simulink model "glideslope_and_flare"  (R2017a)
settings: Solver=VariableStepAuto  StartTime=0.0  StopTime=140  RelTol=1e-3
values from neighbouring files (symbols this model uses):
  A = A_longitude_lo([1,2,3,4,5],[1,2,3,4,5])    [glideslope_and_flare_control.m]
  alpha_trim = trim_state_lin(8)*180/pi    [glideslope_and_flare_control.m]
  B = A_longitude_lo([1,2,3,4,5],[6,7])    [glideslope_and_flare_control.m]
  C = C_longitude_lo([1,2,3,4,5],[1,2,3,4,5])    [glideslope_and_flare_control.m]
  D = C_longitude_lo([1,2,3,4,5],[6,7])    [glideslope_and_flare_control.m]
  glide_slope_ref = 3    [glideslope_and_flare_control.m]
  hf = x2*tan(glide_slope_ref*pi/180)+10    [glideslope_and_flare_control.m]
  ht_trim = trim_state_lin(3)    [glideslope_and_flare_control.m]
  runway_altitude = 3000    [glideslope_and_flare_control.m]
  tau = x1/(flaretouchdowntime*velocity_trim-velocity_trim*cos(glide_slope_ref*pi/180))    [glideslope_and_flare_control.m]
  theta_trim = trim_state_lin(5)*180/pi    [glideslope_and_flare_control.m]
  time_interception = 10    [glideslope_and_flare_control.m]
  trim_control_lin = trim_control_lo    [FindF16Dynamics.m]
  trim_thrust_lin = trim_thrust_lo    [FindF16Dynamics.m]
  velocity_trim = trim_state_lin(7)    [glideslope_and_flare_control.m]
undefined symbols (not defined in the file or in its folder): magnitude
libraries: simulink x8
settings Model: Creator=chatto  LastModifiedBy=chatto

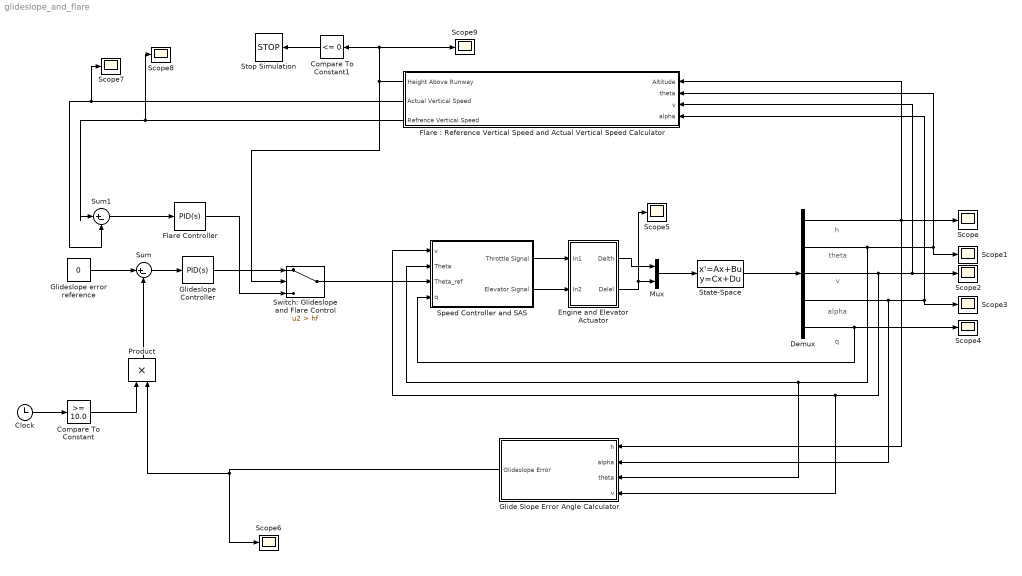
== system glideslope_and_flare ==
  note: alpha
  note: v
  note: theta
  note: h
  note: q
  Clock : Clock
  Compare To Constant : simulink/Logic and Bit Operations/Compare To Constant  relop=>=  const=10.0  OutDataTypeStr=boolean
  Compare To Constant1 : simulink/Logic and Bit Operations/Compare To Constant  relop=<=  const=0  OutDataTypeStr=boolean
  Demux : Demux  Outputs=5
  Engine and Elevator Actuator : Subsystem
  "Flare : Reference Vertical Speed and Actual Vertical Speed Calculator" : Subsystem
  Flare Controller : simulink/Continuous/PID Controller  Controller=PID  TimeDomain=Continuous-time  SampleTime=-1  IntegratorMethod=Forward Euler  FilterMethod=Forward Euler  Form=Parallel  UseFilter=on  ControllerParametersSource=internal  P=0.33  I=0  D=0.33  N=100  InitialConditionSource=internal  InitialConditionForIntegrator=0  InitialConditionForFilter=0  ExternalReset=none  LimitOutput=off  UpperSaturationLimit=inf  LowerSaturationLimit=-inf  LinearizeAsGain=on  AntiWindupMode=none  Kb=1  TrackingMode=off  Kt=1  PParamMin=[]  PParamMax=[]  IParamMin=[]  IParamMax=[]  DParamMin=[]  DParamMax=[]  NParamMin=[]  NParamMax=[]  KbParamMin=[]  KbParamMax=[]  KtParamMin=[]  KtParamMax=[]  POutMin=[]  POutMax=[]  IOutMin=[]  IOutMax=[]  DOutMin=[]  DOutMax=[]  NOutMin=[]  NOutMax=[]  KbOutMin=[]  KbOutMax=[]  KtOutMin=[]  KtOutMax=[]  IntegratorOutMin=[]  IntegratorOutMax=[]  FilterOutMin=[]  FilterOutMax=[]  SumOutMin=[]  SumOutMax=[]  SumI1OutMin=[]  SumI1OutMax=[]  SumI2OutMin=[]  SumI2OutMax=[]  SumI3OutMin=[]  SumI3OutMax=[]  SumDOutMin=[]  SumDOutMax=[]  SaturationOutMin=[]  SaturationOutMax=[]  IntegratorContinuousStateAttributes=''  IntegratorStateMustResolveToSignalObject=off  IntegratorRTWStateStorageClass=Auto  FilterContinuousStateAttributes=''  FilterStateMustResolveToSignalObject=off  FilterRTWStateStorageClass=Auto  DifferentiatorICPrevScaledInput=0  DifferentiatorOutMin=[]  DifferentiatorOutMax=[]  InitialConditionSetting=State (most efficient)
  Glide Slope Error Angle Calculator : Subsystem
  Glideslope Controller : simulink/Continuous/PID Controller  Controller=PID  TimeDomain=Continuous-time  SampleTime=-1  IntegratorMethod=Forward Euler  FilterMethod=Forward Euler  Form=Parallel  UseFilter=on  ControllerParametersSource=internal  P=80  I=8  D=100  N=100  InitialConditionSource=internal  InitialConditionForIntegrator=0  InitialConditionForFilter=0  ExternalReset=none  LimitOutput=off  UpperSaturationLimit=inf  LowerSaturationLimit=-inf  LinearizeAsGain=on  AntiWindupMode=none  Kb=1  TrackingMode=off  Kt=1  PParamMin=[]  PParamMax=[]  IParamMin=[]  IParamMax=[]  DParamMin=[]  DParamMax=[]  NParamMin=[]  NParamMax=[]  KbParamMin=[]  KbParamMax=[]  KtParamMin=[]  KtParamMax=[]  POutMin=[]  POutMax=[]  IOutMin=[]  IOutMax=[]  DOutMin=[]  DOutMax=[]  NOutMin=[]  NOutMax=[]  KbOutMin=[]  KbOutMax=[]  KtOutMin=[]  KtOutMax=[]  IntegratorOutMin=[]  IntegratorOutMax=[]  FilterOutMin=[]  FilterOutMax=[]  SumOutMin=[]  SumOutMax=[]  SumI1OutMin=[]  SumI1OutMax=[]  SumI2OutMin=[]  SumI2OutMax=[]  SumI3OutMin=[]  SumI3OutMax=[]  SumDOutMin=[]  SumDOutMax=[]  SaturationOutMin=[]  SaturationOutMax=[]  IntegratorContinuousStateAttributes=''  IntegratorStateMustResolveToSignalObject=off  IntegratorRTWStateStorageClass=Auto  FilterContinuousStateAttributes=''  FilterStateMustResolveToSignalObject=off  FilterRTWStateStorageClass=Auto  DifferentiatorICPrevScaledInput=0  DifferentiatorOutMin=[]  DifferentiatorOutMax=[]  InitialConditionSetting=State (most efficient)
  Glideslope error reference : Constant  Value=0
  Mux : Mux  Inputs=2
  Product : Product
  Scope{,1..9} (10 alike) : Scope
  Speed Controller and SAS : Subsystem
  State-Space : StateSpace  A=A  B=B  C=C  D=D  X0=0
  Stop Simulation : Stop
  Sum : Sum  Inputs=|+-
  Sum1 : Sum  Inputs=|+-
  Switch: Glideslope and Flare Control : Switch  Criteria=u2 > Threshold  Threshold=hf
  wires:
  Mux/1 -> State-Space/1
  State-Space/1 -> Demux/1
  Engine and Elevator Actuator/1(Delth) -> Mux/1
  Engine and Elevator Actuator/2(Delel) -> Scope5/1, Mux/2
  Sum/1 -> Glideslope Controller/1
  Speed Controller and SAS/1(Throttle Signal) -> Engine and Elevator Actuator/1(In1)
  Speed Controller and SAS/2(Elevator Signal) -> Engine and Elevator Actuator/2(In2)
  Demux/5 -> Speed Controller and SAS/4(q), Scope4/1
  Glideslope error reference/1 -> Sum/1
  Glideslope Controller/1 -> Switch: Glideslope and Flare Control/1
  Clock/1 -> Compare To Constant/1
  Compare To Constant/1 -> Product/1
  Product/1 -> Sum/2
  Glide Slope Error Angle Calculator/1(Glideslope Error) -> Scope6/1, Product/2
  Demux/1 -> Glide Slope Error Angle Calculator/1(h), Scope/1, "Flare : Reference Vertical Speed and Actual Vertical Speed Calculator"/1(Altitude)
  Demux/3 -> "Flare : Reference Vertical Speed and Actual Vertical Speed Calculator"/3(v), Scope2/1, Glide Slope Error Angle Calculator/4(v), Speed Controller and SAS/1(v)
  Demux/2 -> "Flare : Reference Vertical Speed and Actual Vertical Speed Calculator"/2(theta), Scope1/1, Glide Slope Error Angle Calculator/3(theta), Speed Controller and SAS/2(Theta)
  Demux/4 -> Glide Slope Error Angle Calculator/2(alpha), "Flare : Reference Vertical Speed and Actual Vertical Speed Calculator"/4(alpha), Scope3/1
  "Flare : Reference Vertical Speed and Actual Vertical Speed Calculator"/3(Refrence Vertical Speed) -> Scope8/1, Sum1/1
  "Flare : Reference Vertical Speed and Actual Vertical Speed Calculator"/2(Actual Vertical Speed) -> Scope7/1, Sum1/2
  Compare To Constant1/1 -> Stop Simulation/1
  Sum1/1 -> Flare Controller/1
  Switch: Glideslope and Flare Control/1 -> Speed Controller and SAS/3(Theta_ref)
  Flare Controller/1 -> Switch: Glideslope and Flare Control/3
  "Flare : Reference Vertical Speed and Actual Vertical Speed Calculator"/1(Height Above Runway) -> Scope9/1, Compare To Constant1/1, Switch: Glideslope and Flare Control/2

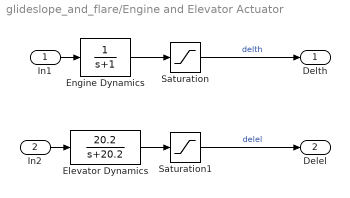
== system glideslope_and_flare/Engine and Elevator Actuator ==
  In1 : Inport
  In2 : Inport  Port=2
  Elevator Dynamics : TransferFcn  Numerator=[20.2]  Denominator=[1 20.2]
  Engine Dynamics : TransferFcn  Denominator=[1 1]
  Saturation : Saturate  UpperLimit=19000-trim_thrust_lin  LowerLimit=1000-trim_thrust_lin
  Saturation1 : Saturate  UpperLimit=25-trim_control_lin(1)  LowerLimit=-25-trim_control_lin(1)
  Delth : Outport
  Delel : Outport  Port=2
  wires:
  Saturation1/1 -> Delel/1  "delel"
  In1/1 -> Engine Dynamics/1
  In2/1 -> Elevator Dynamics/1
  Elevator Dynamics/1 -> Saturation1/1
  Engine Dynamics/1 -> Saturation/1
  Saturation/1 -> Delth/1  "delth"

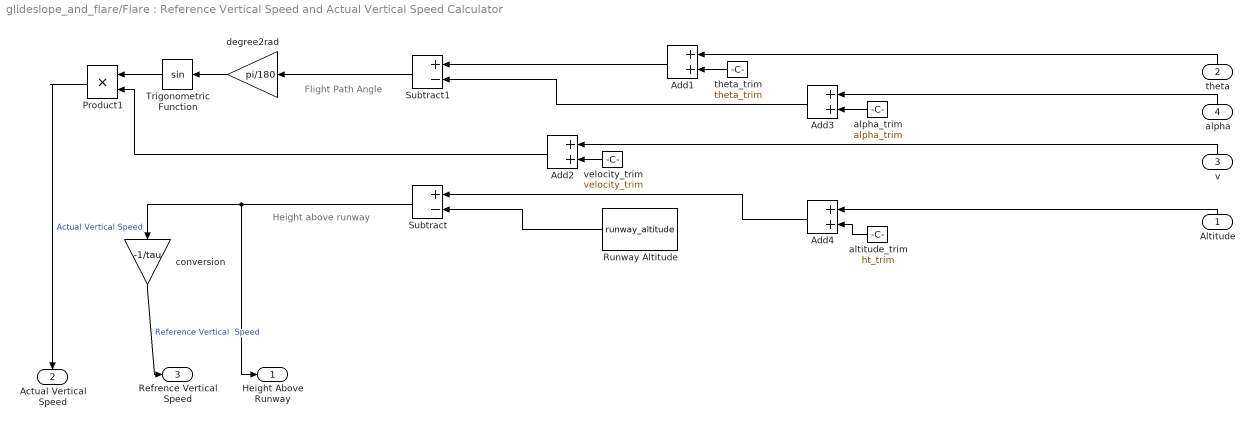
== system glideslope_and_flare/Flare : Reference Vertical Speed and Actual Vertical Speed Calculator ==
  note: Flight Path Angle
  note: Height above runway
  Altitude : Inport
  theta : Inport  Port=2
  v : Inport  Port=3
  alpha : Inport  Port=4
  Add{1..4} (4 alike) : Sum
  Product1 : Product
  Runway Altitude : Constant  Value=runway_altitude
  Subtract : Sum  Inputs=+-
  Subtract1 : Sum  Inputs=+-
  Trigonometric Function : Trigonometry
  alpha_trim : Constant  Value=alpha_trim
  altitude_trim : Constant  Value=ht_trim
  conversion : Gain  Gain=-1/tau
  degree2rad : Gain  Gain=pi/180
  theta_trim : Constant  Value=theta_trim
  velocity_trim : Constant  Value=velocity_trim
  Height Above Runway : Outport
  Actual Vertical Speed : Outport  Port=2
  Refrence Vertical Speed : Outport  Port=3
  wires:
  alpha_trim/1 -> Add3/2
  Runway Altitude/1 -> Subtract/2
  Trigonometric Function/1 -> Product1/1
  Altitude/1 -> Add4/1
  Add4/1 -> Subtract/1
  Add3/1 -> Subtract1/2
  alpha/1 -> Add3/1
  theta/1 -> Add1/1
  Product1/1 -> Actual Vertical Speed/1  "Actual Vertical Speed"
  theta_trim/1 -> Add1/2
  degree2rad/1 -> Trigonometric Function/1
  Add2/1 -> Product1/2
  v/1 -> Add2/1
  Add1/1 -> Subtract1/1
  altitude_trim/1 -> Add4/2
  conversion/1 -> Refrence Vertical Speed/1  "Reference Vertical  Speed"
  Subtract1/1 -> degree2rad/1
  velocity_trim/1 -> Add2/2
  Subtract/1 -> Height Above Runway/1, conversion/1

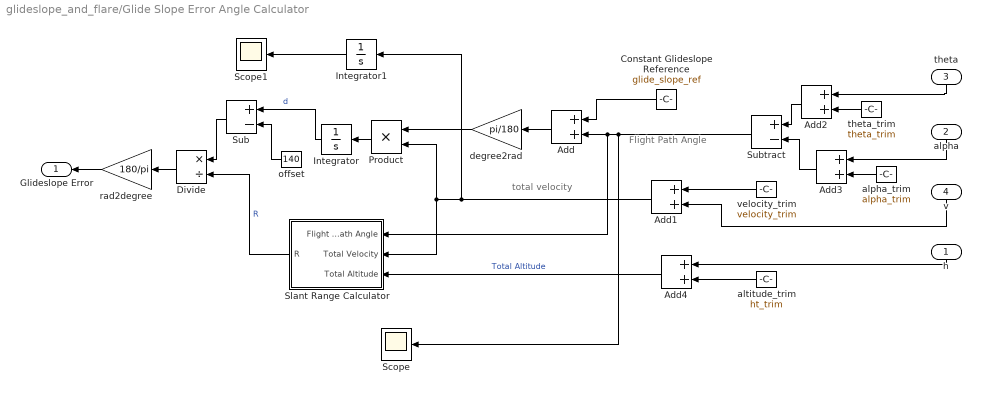
== system glideslope_and_flare/Glide Slope Error Angle Calculator ==
  note: total velocity
  note: Flight Path Angle
  h : Inport
  alpha : Inport  Port=2
  theta : Inport  Port=3
  v : Inport  Port=4
  Add{,1..4} (5 alike) : Sum
  Constant Glideslope Reference : Constant  Value=glide_slope_ref
  Divide : Product  Inputs=*/
  Integrator : Integrator
  Integrator1 : Integrator
  Product : Product
  Scope : Scope
  Scope1 : Scope
  Slant Range Calculator : Subsystem
  Sub : Sum  Inputs=+-
  Subtract : Sum  Inputs=+-
  alpha_trim : Constant  Value=alpha_trim
  altitude_trim : Constant  Value=ht_trim
  degree2rad : Gain  Gain=pi/180
  offset : Constant  Value=140
  rad2degree : Gain  Gain=180/pi
  theta_trim : Constant  Value=theta_trim
  velocity_trim : Constant  Value=velocity_trim
  Glideslope Error : Outport
  wires:
  altitude_trim/1 -> Add4/2
  Divide/1 -> rad2degree/1
  velocity_trim/1 -> Add1/1
  v/1 -> Add1/2
  alpha_trim/1 -> Add3/2
  Add2/1 -> Subtract/1
  theta_trim/1 -> Add2/2
  Add4/1 -> Slant Range Calculator/3(Total Altitude)  "Total Altitude"
  Constant Glideslope Reference/1 -> Add/1
  alpha/1 -> Add3/1
  h/1 -> Add4/1
  theta/1 -> Add2/1
  Add/1 -> degree2rad/1
  Add3/1 -> Subtract/2
  Integrator/1 -> Sub/1  "d"
  degree2rad/1 -> Product/1
  Product/1 -> Integrator/1
  Slant Range Calculator/1(R) -> Divide/2  "R"
  rad2degree/1 -> Glideslope Error/1
  Add1/1 -> Integrator1/1, Product/2, Slant Range Calculator/2(Total Velocity)
  Subtract/1 -> Slant Range Calculator/1(Flight Path Angle), Add/2, Scope/1
  offset/1 -> Sub/2
  Sub/1 -> Divide/1
  Integrator1/1 -> Scope1/1

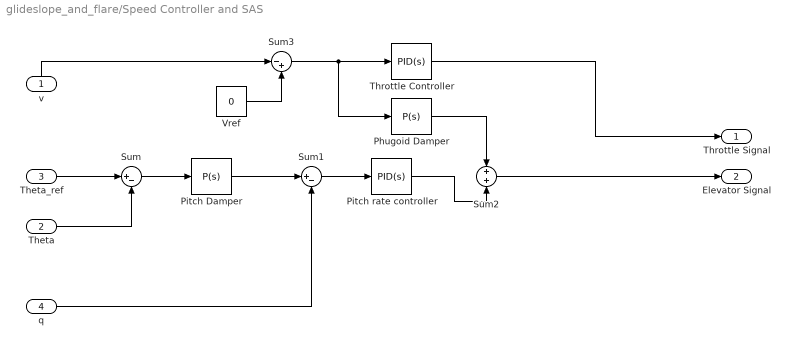
== system glideslope_and_flare/Speed Controller and SAS ==
  v : Inport
  Theta : Inport  Port=2
  Theta_ref : Inport  Port=3
  q : Inport  Port=4
  Phugoid Damper : simulink/Continuous/PID Controller  Controller=P  TimeDomain=Continuous-time  SampleTime=-1  IntegratorMethod=Forward Euler  FilterMethod=Forward Euler  Form=Parallel  UseFilter=on  ControllerParametersSource=internal  P=0.05  I=0.001  D=0.5  N=100  InitialConditionSource=internal  InitialConditionForIntegrator=0  InitialConditionForFilter=0  ExternalReset=none  LimitOutput=off  UpperSaturationLimit=inf  LowerSaturationLimit=-inf  LinearizeAsGain=on  AntiWindupMode=none  Kb=1  TrackingMode=off  Kt=1  PParamMin=[]  PParamMax=[]  IParamMin=[]  IParamMax=[]  DParamMin=[]  DParamMax=[]  NParamMin=[]  NParamMax=[]  KbParamMin=[]  KbParamMax=[]  KtParamMin=[]  KtParamMax=[]  POutMin=[]  POutMax=[]  IOutMin=[]  IOutMax=[]  DOutMin=[]  DOutMax=[]  NOutMin=[]  NOutMax=[]  KbOutMin=[]  KbOutMax=[]  KtOutMin=[]  KtOutMax=[]  IntegratorOutMin=[]  IntegratorOutMax=[]  FilterOutMin=[]  FilterOutMax=[]  SumOutMin=[]  SumOutMax=[]  SumI1OutMin=[]  SumI1OutMax=[]  SumI2OutMin=[]  SumI2OutMax=[]  SumI3OutMin=[]  SumI3OutMax=[]  SumDOutMin=[]  SumDOutMax=[]  SaturationOutMin=[]  SaturationOutMax=[]  IntegratorContinuousStateAttributes=''  IntegratorStateMustResolveToSignalObject=off  IntegratorRTWStateStorageClass=Auto  FilterContinuousStateAttributes=''  FilterStateMustResolveToSignalObject=off  FilterRTWStateStorageClass=Auto  DifferentiatorICPrevScaledInput=0  DifferentiatorOutMin=[]  DifferentiatorOutMax=[]  InitialConditionSetting=State (most efficient)
  Pitch Damper : simulink/Continuous/PID Controller  Controller=P  TimeDomain=Continuous-time  SampleTime=-1  IntegratorMethod=Forward Euler  FilterMethod=Forward Euler  Form=Parallel  UseFilter=on  ControllerParametersSource=internal  P=0.5  I=0  D=0  N=100  InitialConditionSource=internal  InitialConditionForIntegrator=0  InitialConditionForFilter=0  ExternalReset=none  LimitOutput=off  UpperSaturationLimit=inf  LowerSaturationLimit=-inf  LinearizeAsGain=on  AntiWindupMode=none  Kb=1  TrackingMode=off  Kt=1  PParamMin=[]  PParamMax=[]  IParamMin=[]  IParamMax=[]  DParamMin=[]  DParamMax=[]  NParamMin=[]  NParamMax=[]  KbParamMin=[]  KbParamMax=[]  KtParamMin=[]  KtParamMax=[]  POutMin=[]  POutMax=[]  IOutMin=[]  IOutMax=[]  DOutMin=[]  DOutMax=[]  NOutMin=[]  NOutMax=[]  KbOutMin=[]  KbOutMax=[]  KtOutMin=[]  KtOutMax=[]  IntegratorOutMin=[]  IntegratorOutMax=[]  FilterOutMin=[]  FilterOutMax=[]  SumOutMin=[]  SumOutMax=[]  SumI1OutMin=[]  SumI1OutMax=[]  SumI2OutMin=[]  SumI2OutMax=[]  SumI3OutMin=[]  SumI3OutMax=[]  SumDOutMin=[]  SumDOutMax=[]  SaturationOutMin=[]  SaturationOutMax=[]  IntegratorContinuousStateAttributes=''  IntegratorStateMustResolveToSignalObject=off  IntegratorRTWStateStorageClass=Auto  FilterContinuousStateAttributes=''  FilterStateMustResolveToSignalObject=off  FilterRTWStateStorageClass=Auto  DifferentiatorICPrevScaledInput=0  DifferentiatorOutMin=[]  DifferentiatorOutMax=[]  InitialConditionSetting=State (most efficient)
  Pitch rate controller : simulink/Continuous/PID Controller  Controller=PID  TimeDomain=Continuous-time  SampleTime=-1  IntegratorMethod=Forward Euler  FilterMethod=Forward Euler  Form=Parallel  UseFilter=on  ControllerParametersSource=internal  P=-5  I=-15  D=-0.5  N=100  InitialConditionSource=internal  InitialConditionForIntegrator=0  InitialConditionForFilter=0  ExternalReset=none  LimitOutput=off  UpperSaturationLimit=inf  LowerSaturationLimit=-inf  LinearizeAsGain=on  AntiWindupMode=none  Kb=1  TrackingMode=off  Kt=1  PParamMin=[]  PParamMax=[]  IParamMin=[]  IParamMax=[]  DParamMin=[]  DParamMax=[]  NParamMin=[]  NParamMax=[]  KbParamMin=[]  KbParamMax=[]  KtParamMin=[]  KtParamMax=[]  POutMin=[]  POutMax=[]  IOutMin=[]  IOutMax=[]  DOutMin=[]  DOutMax=[]  NOutMin=[]  NOutMax=[]  KbOutMin=[]  KbOutMax=[]  KtOutMin=[]  KtOutMax=[]  IntegratorOutMin=[]  IntegratorOutMax=[]  FilterOutMin=[]  FilterOutMax=[]  SumOutMin=[]  SumOutMax=[]  SumI1OutMin=[]  SumI1OutMax=[]  SumI2OutMin=[]  SumI2OutMax=[]  SumI3OutMin=[]  SumI3OutMax=[]  SumDOutMin=[]  SumDOutMax=[]  SaturationOutMin=[]  SaturationOutMax=[]  IntegratorContinuousStateAttributes=''  IntegratorStateMustResolveToSignalObject=off  IntegratorRTWStateStorageClass=Auto  FilterContinuousStateAttributes=''  FilterStateMustResolveToSignalObject=off  FilterRTWStateStorageClass=Auto  DifferentiatorICPrevScaledInput=0  DifferentiatorOutMin=[]  DifferentiatorOutMax=[]  InitialConditionSetting=State (most efficient)
  Sum : Sum  Inputs=|+-
  Sum1 : Sum  Inputs=|+-
  Sum2 : Sum
  Sum3 : Sum  Inputs=|-+
  Throttle Controller : simulink/Continuous/PID Controller  Controller=PID  TimeDomain=Continuous-time  SampleTime=-1  IntegratorMethod=Forward Euler  FilterMethod=Forward Euler  Form=Parallel  UseFilter=on  ControllerParametersSource=internal  P=8000  I=10  D=10000  N=100  InitialConditionSource=internal  InitialConditionForIntegrator=0  InitialConditionForFilter=0  ExternalReset=none  LimitOutput=off  UpperSaturationLimit=inf  LowerSaturationLimit=-inf  LinearizeAsGain=on  AntiWindupMode=none  Kb=1  TrackingMode=off  Kt=1  PParamMin=[]  PParamMax=[]  IParamMin=[]  IParamMax=[]  DParamMin=[]  DParamMax=[]  NParamMin=[]  NParamMax=[]  KbParamMin=[]  KbParamMax=[]  KtParamMin=[]  KtParamMax=[]  POutMin=[]  POutMax=[]  IOutMin=[]  IOutMax=[]  DOutMin=[]  DOutMax=[]  NOutMin=[]  NOutMax=[]  KbOutMin=[]  KbOutMax=[]  KtOutMin=[]  KtOutMax=[]  IntegratorOutMin=[]  IntegratorOutMax=[]  FilterOutMin=[]  FilterOutMax=[]  SumOutMin=[]  SumOutMax=[]  SumI1OutMin=[]  SumI1OutMax=[]  SumI2OutMin=[]  SumI2OutMax=[]  SumI3OutMin=[]  SumI3OutMax=[]  SumDOutMin=[]  SumDOutMax=[]  SaturationOutMin=[]  SaturationOutMax=[]  IntegratorContinuousStateAttributes=''  IntegratorStateMustResolveToSignalObject=off  IntegratorRTWStateStorageClass=Auto  FilterContinuousStateAttributes=''  FilterStateMustResolveToSignalObject=off  FilterRTWStateStorageClass=Auto  DifferentiatorICPrevScaledInput=0  DifferentiatorOutMin=[]  DifferentiatorOutMax=[]  InitialConditionSetting=State (most efficient)
  Vref : Constant  Value=0
  Throttle Signal : Outport
  Elevator Signal : Outport  Port=2
  wires:
  Theta/1 -> Sum/2
  Vref/1 -> Sum3/2
  Phugoid Damper/1 -> Sum2/1
  Pitch Damper/1 -> Sum1/1
  v/1 -> Sum3/1
  q/1 -> Sum1/2
  Sum2/1 -> Elevator Signal/1
  Theta_ref/1 -> Sum/1
  Sum3/1 -> Phugoid Damper/1, Throttle Controller/1
  Sum1/1 -> Pitch rate controller/1
  Sum/1 -> Pitch Damper/1
  Throttle Controller/1 -> Throttle Signal/1
  Pitch rate controller/1 -> Sum2/2

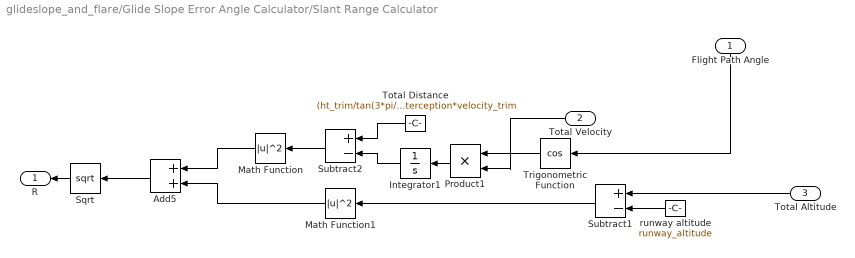
== system glideslope_and_flare/Glide Slope Error Angle Calculator/Slant Range Calculator ==
  Flight Path Angle : Inport
  Total Velocity : Inport  Port=2
  Total Altitude : Inport  Port=3
  Add5 : Sum
  Integrator1 : Integrator
  Math Function : Math  Operator=magnitude^2  SaturateOnIntegerOverflow=on
  Math Function1 : Math  Operator=magnitude^2  SaturateOnIntegerOverflow=on
  Product1 : Product
  Sqrt : Sqrt  SaturateOnIntegerOverflow=on
  Subtract1 : Sum  Inputs=+-
  Subtract2 : Sum  Inputs=+-
  "Total Distance " : Constant  Value=(ht_trim/tan(3*pi/180))+time_interception*velocity_trim
  Trigonometric Function : Trigonometry  Operator=cos
  runway altitude : Constant  Value=runway_altitude
  R : Outport
  wires:
  Subtract2/1 -> Math Function/1
  runway altitude/1 -> Subtract1/2
  Total Altitude/1 -> Subtract1/1
  Trigonometric Function/1 -> Product1/1
  "Total Distance "/1 -> Subtract2/1
  Subtract1/1 -> Math Function1/1
  Integrator1/1 -> Subtract2/2
  Math Function/1 -> Add5/1
  Add5/1 -> Sqrt/1
  Flight Path Angle/1 -> Trigonometric Function/1
  Product1/1 -> Integrator1/1
  Sqrt/1 -> R/1
  Math Function1/1 -> Add5/2
  Total Velocity/1 -> Product1/2
